simulink model "DTU_Topology_Medium_Line"  (R2023b)
settings: Solver=ode4  StartTime=0.0  StopTime=stoptime  FixedStep=Ts  RelTol=1e-3
PreLoadFcn:
  | Ts=1e-4;run('Grid_Parameters_3ph.m');load('Data_3ph_Pars.mat');load('First_Busbar_Pars.mat');load('PV_Busbar_Pars.mat');load('V2G_Busbar_Pars.mat');run('line_parameters.m')
PostLoadFcn:
  | Ts=1e-4;run('Grid_Parameters_3ph.m');load('Data_3ph_Pars.mat');load('First_Busbar_Pars.mat');load('PV_Busbar_Pars.mat');load('V2G_Busbar_Pars.mat');run('line_parameters.m')
InitFcn:
  | Ts=1e-4;run('Grid_Parameters_3ph.m');load('Data_3ph_Pars.mat');load('First_Busbar_Pars.mat');load('PV_Busbar_Pars.mat');load('V2G_Busbar_Pars.mat');run('line_parameters.m')
StartFcn:
  | Ts=1e-4;run('Grid_Parameters_3ph.m');load('Data_3ph_Pars.mat');load('First_Busbar_Pars.mat');load('PV_Busbar_Pars.mat');load('V2G_Busbar_Pars.mat');run('line_parameters.m')
values from neighbouring files (symbols this model uses):
  datastart = 6100    [Grid_Parameters_3ph.m]
  datastop = 6300    [Grid_Parameters_3ph.m]
  fnom = 50    [Grid_Parameters_3ph.m]    (also in line_parameters.m)
  line_param = struct()    [line_parameters.m]
  t_factor = 1/acceleration    (= 1)    [Grid_Parameters_3ph.m]
  timestep_meas_data = 1    [Grid_Parameters_3ph.m]
  Vnom = 400    [Grid_Parameters_3ph.m]
undefined symbols (not defined in the file or in its folder): another_event_name, Data_3ph_Pars, j, my_event_name, Newton, PV_Busbar_Pars, Raphson, V2G_Busbar_Pars
libraries: spsSeriesRLCBranchLib x57, spsGroundLib x30, spsThreePhaseVIMeasurementLib x17, spsControlledCurrentSourceLib x9, spsThreePhaseSineGeneratorLib x9, spsMeanLib x7, spsMutualInductanceLib x4, rtlab x2, spsThreePhaseSourceLib x1, sps_lib x1
(part 2 of 2)

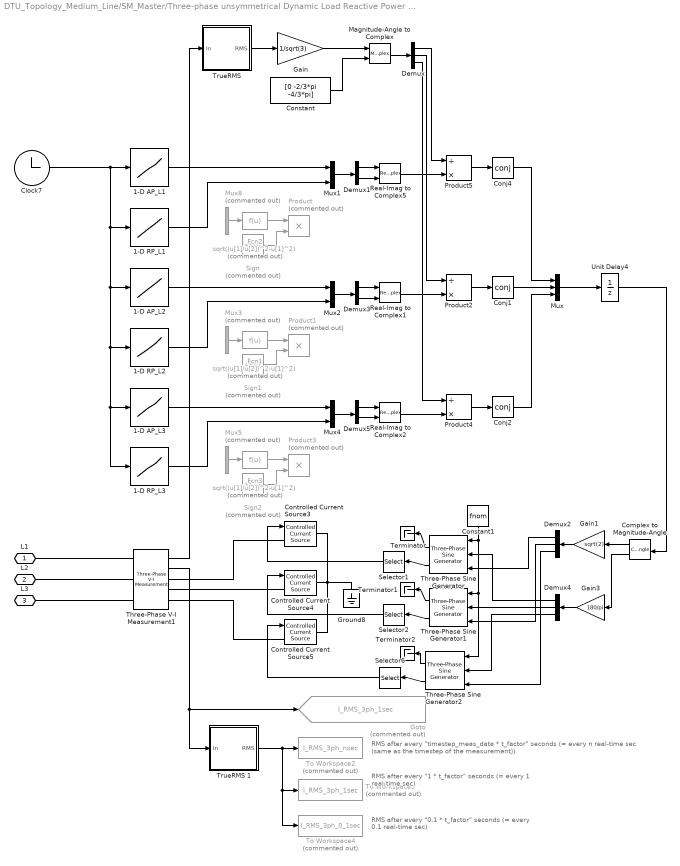
== system DTU_Topology_Medium_Line/SM_Master/Three-phase unsymmetrical Dynamic Load Reactive Power input PV ==
  note: RMS after every "1 * t_factor" seconds
      | (= every 1 real-time sec)
  note: RMS after every "0.1 * t_factor" seconds
      | (= every 0.1 real-time sec)
  note: RMS after every "timestep_meas_data * t_factor" seconds
      | (= every n real-time sec (same as the timestep of the measurement))
  1-D AP_L1 : Lookup_n-D  NumberOfTableDimensions=1  BreakpointsForDimension1=t_factor * [0:timestep_meas_data:(PV_Busbar_Pars.Time(datastop)-PV_Busbar_Pars.Time(datastart))]'  Table=PV_Busbar_Pars.ActivePowerL1(datastart:datastop)  InterpMethod=Flat  InternalRulePriority=Speed  RndMeth=Simplest
  1-D AP_L2 : Lookup_n-D  NumberOfTableDimensions=1  BreakpointsForDimension1=t_factor * [0:timestep_meas_data:(PV_Busbar_Pars.Time(datastop)-PV_Busbar_Pars.Time(datastart))]'  Table=PV_Busbar_Pars.ActivePowerL2(datastart:datastop)  InterpMethod=Flat  InternalRulePriority=Speed  RndMeth=Simplest
  1-D AP_L3 : Lookup_n-D  NumberOfTableDimensions=1  BreakpointsForDimension1=t_factor * [0:timestep_meas_data:(PV_Busbar_Pars.Time(datastop)-PV_Busbar_Pars.Time(datastart))]'  Table=PV_Busbar_Pars.ActivePowerL3(datastart:datastop)  InterpMethod=Flat  InternalRulePriority=Speed  RndMeth=Simplest
  1-D RP_L1 : Lookup_n-D  NumberOfTableDimensions=1  BreakpointsForDimension1=t_factor * [0:timestep_meas_data:(PV_Busbar_Pars.Time(datastop)-PV_Busbar_Pars.Time(datastart))]'  Table=PV_Busbar_Pars.ReactivePowerL1(datastart:datastop)  InterpMethod=Flat  InternalRulePriority=Speed  RndMeth=Simplest
  1-D RP_L2 : Lookup_n-D  NumberOfTableDimensions=1  BreakpointsForDimension1=t_factor * [0:timestep_meas_data:(PV_Busbar_Pars.Time(datastop)-PV_Busbar_Pars.Time(datastart))]'  Table=PV_Busbar_Pars.ReactivePowerL2(datastart:datastop)  InterpMethod=Flat  InternalRulePriority=Speed  RndMeth=Simplest
  1-D RP_L3 : Lookup_n-D  NumberOfTableDimensions=1  BreakpointsForDimension1=t_factor * [0:timestep_meas_data:(PV_Busbar_Pars.Time(datastop)-PV_Busbar_Pars.Time(datastart))]'  Table=PV_Busbar_Pars.ReactivePowerL3(datastart:datastop)  InterpMethod=Flat  InternalRulePriority=Speed  RndMeth=Simplest
  Clock7 : Clock
  Complex to Magnitude-Angle : ComplexToMagnitudeAngle
  Conj1 : Math  Operator=conj  SignedPower=on
  Conj2 : Math  Operator=conj  SignedPower=on
  Conj4 : Math  Operator=conj  SignedPower=on
  Constant : Constant  Value=[0 -2/3*pi -4/3*pi]
  Constant1 : Constant  Value=fnom
  Controlled Current Source3 : spsControlledCurrentSourceLib/Controlled Current Source  Initialize=on  Source_Type=AC  Amplitude=0  Phase=0  Frequency=50  Measurements=Current
  Controlled Current Source4 : spsControlledCurrentSourceLib/Controlled Current Source  Initialize=on  Source_Type=AC  Amplitude=0  Phase=0  Frequency=50  Measurements=Current
  Controlled Current Source5 : spsControlledCurrentSourceLib/Controlled Current Source  Initialize=on  Source_Type=AC  Amplitude=0  Phase=0  Frequency=50  Measurements=Current
  Demux : Demux  Outputs=3
  Demux1 : Demux  Outputs=2
      settings: DisplayOption=none
  Demux2 : Demux  Outputs=3
  Demux3 : Demux  Outputs=2
      settings: DisplayOption=none
  Demux4 : Demux  Outputs=3
  Demux5 : Demux  Outputs=2
      settings: DisplayOption=none
  Fcn1 : Fcn  Commented=on  Expr=sqrt((u[1]/u[2])^2-u[1]^2)
  Fcn2 : Fcn  Commented=on  Expr=sqrt((u[1]/u[2])^2-u[1]^2)
  Fcn3 : Fcn  Commented=on  Expr=sqrt((u[1]/u[2])^2-u[1]^2)
  Gain : Gain  Gain=1/sqrt(3)
  Gain1 : Gain  Gain=sqrt(2)
  Gain3 : Gain  Gain=180/pi
  Goto : Goto  Commented=on  GotoTag=I_RMS_3ph_1sec  TagVisibility=global
  Ground8 : spsGroundLib/Ground  LConnTagsString=a
  Magnitude-Angle to Complex : MagnitudeAngleToComplex
  Mux : Mux  Inputs=3
  Mux1 : Mux  Inputs=2
  Mux2 : Mux  Inputs=2
  Mux3 : Mux  Commented=on  Inputs=2
  Mux4 : Mux  Inputs=2
  Mux5 : Mux  Commented=on  Inputs=2
  Mux8 : Mux  Commented=on  Inputs=2
  Product : Product  Commented=on
  Product1 : Product  Commented=on
  Product2 : Product  Inputs=/*  InputSameDT=on  SaturateOnIntegerOverflow=on  OutDataTypeStr=Inherit: Same as first input
  Product3 : Product  Commented=on
  Product4 : Product  Inputs=/*  InputSameDT=on  SaturateOnIntegerOverflow=on  OutDataTypeStr=Inherit: Same as first input
  Product5 : Product  Inputs=/*  InputSameDT=on  SaturateOnIntegerOverflow=on  OutDataTypeStr=Inherit: Same as first input
  Real-Imag to Complex1 : RealImagToComplex
  Real-Imag to Complex2 : RealImagToComplex
  Real-Imag to Complex5 : RealImagToComplex
  Selector1 : Selector  InputPortWidth=3  IndexOptions=Index vector (dialog)  Indices=1  OutputSizes=1
  Selector2 : Selector  InputPortWidth=3  IndexOptions=Index vector (dialog)  Indices=1  OutputSizes=1
  Selector6 : Selector  InputPortWidth=3  IndexOptions=Index vector (dialog)  Indices=1  OutputSizes=1
  Sign : Signum  Commented=on
  Sign1 : Signum  Commented=on
  Sign2 : Signum  Commented=on
  Terminator : Terminator
  Terminator1 : Terminator
  Terminator2 : Terminator
  Three-Phase Sine Generator : spsThreePhaseSineGeneratorLib/Three-Phase Sine Generator  Ts=0
      settings: LibrarySourceBlock=|
      | sps_lib/Sources/Signal Generator Sources/Three-Phase
      | Sine Generator
  Three-Phase Sine Generator1 : spsThreePhaseSineGeneratorLib/Three-Phase Sine Generator  Ts=0
      settings: LibrarySourceBlock=|
      | sps_lib/Sources/Signal Generator Sources/Three-Phase
      | Sine Generator
  Three-Phase Sine Generator2 : spsThreePhaseSineGeneratorLib/Three-Phase Sine Generator  Ts=0
      settings: LibrarySourceBlock=|
      | sps_lib/Sources/Signal Generator Sources/Three-Phase
      | Sine Generator
  Three-Phase V-I Measurement1 : spsThreePhaseVIMeasurementLib/Three-Phase V-I Measurement  VoltageMeasurement=phase-to-phase  SetLabelV=off  LabelV=Vabc  Vpu=off  VpuLL=off  CurrentMeasurement=yes  SetLabelI=off  LabelI=Iabc  Ipu=off  Pbase=100e6  Vbase=Vnom*sqrt(3)  OutputType=Complex  PhasorSimulation=off  PSBequivalent=0
  To Workspace2 : ToWorkspace  Commented=on  VariableName=I_RMS_3ph_nsec  SampleTime=timestep_meas_data * t_factor
  To Workspace4 : ToWorkspace  Commented=on  VariableName=I_RMS_3ph_0_1sec  SampleTime=0.1 * t_factor
  To Workspace5 : ToWorkspace  Commented=on  VariableName=I_RMS_3ph_1sec  SampleTime=1 * t_factor
  "TrueRMS " : Subsystem  AncestorBlock=powerlib_meascontrol/Measurements/RMS/TrueRMS
  TrueRMS 1 : Subsystem  AncestorBlock=powerlib_meascontrol/Measurements/RMS/TrueRMS
  Unit Delay4 : UnitDelay  InitialCondition=0*exp(-j*0*pi/180)  SampleTime=Ts  HasFrameUpgradeWarning=on
  L1 : PMIOPort  Side=Right
  L2 : PMIOPort  Port=2  Side=Right
  L3 : PMIOPort  Port=3  Side=Right
  wires:
  1-D AP_L1/1 -> Mux1/1
  Product5/1 -> Conj4/1
  Fcn2/1 -> Product/1
  Three-Phase V-I Measurement1/2 -> Goto/1, TrueRMS 1/1(In)
  Mux1/1 -> Demux1/1
  Real-Imag to Complex5/1 -> Product5/2
  Clock7/1 -> 1-D RP_L1/1, 1-D RP_L2/1, 1-D AP_L3/1, 1-D RP_L3/1, 1-D AP_L2/1, 1-D AP_L1/1
  Sign/1 -> Product/2
  Mux8/1 -> Fcn2/1
  TrueRMS 1/1(RMS) -> To Workspace2/1, To Workspace5/1, To Workspace4/1
  Constant/1 -> Magnitude-Angle to Complex/2
  Demux/1 -> Product5/1
  Demux/2 -> Product2/1
  Demux/3 -> Product4/1
  Magnitude-Angle to Complex/1 -> Demux/1
  Gain/1 -> Magnitude-Angle to Complex/1
  Mux/1 -> Unit Delay4/1
  Complex to Magnitude-Angle/1 -> Gain1/1
  Three-Phase Sine Generator/1 -> Selector1/1
  Three-Phase Sine Generator1/1 -> Selector2/1
  Three-Phase Sine Generator2/1 -> Selector6/1
  Selector2/1 -> Controlled Current Source4/1
  Selector6/1 -> Controlled Current Source5/1
  Demux2/1 -> Three-Phase Sine Generator/1
  Demux2/2 -> Three-Phase Sine Generator1/1
  Demux2/3 -> Three-Phase Sine Generator2/1
  Conj4/1 -> Mux/1
  Conj1/1 -> Mux/2
  Conj2/1 -> Mux/3
  Constant1/1 -> Three-Phase Sine Generator/3, Three-Phase Sine Generator2/3, Three-Phase Sine Generator1/3
  Complex to Magnitude-Angle/2 -> Gain3/1
  Gain3/1 -> Demux4/1
  Selector1/1 -> Controlled Current Source3/1
  Demux4/1 -> Three-Phase Sine Generator/2
  Demux4/2 -> Three-Phase Sine Generator1/2
  Demux4/3 -> Three-Phase Sine Generator2/2
  Gain1/1 -> Demux2/1
  Demux1/1 -> Real-Imag to Complex5/1
  Demux1/2 -> Real-Imag to Complex5/2
  "TrueRMS "/1(RMS) -> Gain/1
  Three-Phase V-I Measurement1/1 -> "TrueRMS "/1(In)
  Unit Delay4/1 -> Complex to Magnitude-Angle/1
  Mux2/1 -> Demux3/1
  Demux3/2 -> Real-Imag to Complex1/2
  Real-Imag to Complex1/1 -> Product2/2
  Sign1/1 -> Product1/2
  Demux3/1 -> Real-Imag to Complex1/1
  Mux3/1 -> Fcn1/1
  1-D AP_L2/1 -> Mux2/1
  Product2/1 -> Conj1/1
  Fcn1/1 -> Product1/1
  Mux4/1 -> Demux5/1
  Demux5/2 -> Real-Imag to Complex2/2
  Real-Imag to Complex2/1 -> Product4/2
  Sign2/1 -> Product3/2
  Demux5/1 -> Real-Imag to Complex2/1
  Mux5/1 -> Fcn3/1
  1-D AP_L3/1 -> Mux4/1
  Product4/1 -> Conj2/1
  Fcn3/1 -> Product3/1
  1-D RP_L1/1 -> Mux1/2
  1-D RP_L2/1 -> Mux2/2
  1-D RP_L3/1 -> Mux4/2
  Three-Phase Sine Generator/2 -> Terminator/1
  Three-Phase Sine Generator1/2 -> Terminator1/1
  Three-Phase Sine Generator2/2 -> Terminator2/1
  connections:
  Three-Phase V-I Measurement1/RConn2 -- Controlled Current Source4/LConn1
  Three-Phase V-I Measurement1/RConn1 -- Controlled Current Source3/LConn1
  Three-Phase V-I Measurement1/RConn3 -- Controlled Current Source5/LConn1
  Controlled Current Source3/RConn1 -- Controlled Current Source4/RConn1 -- Ground8/LConn1 -- Controlled Current Source5/RConn1
  L1/RConn1 -- Three-Phase V-I Measurement1/LConn1
  Three-Phase V-I Measurement1/LConn2 -- L2/RConn1
  Three-Phase V-I Measurement1/LConn3 -- L3/RConn1

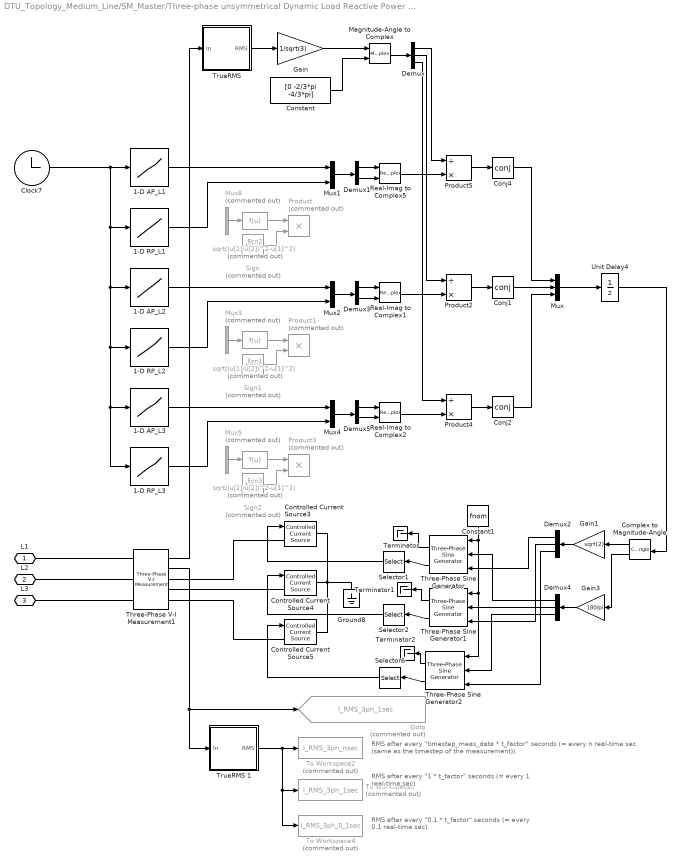
== system DTU_Topology_Medium_Line/SM_Master/Three-phase unsymmetrical Dynamic Load Reactive Power input V2G ==
  note: RMS after every "1 * t_factor" seconds
      | (= every 1 real-time sec)
  note: RMS after every "0.1 * t_factor" seconds
      | (= every 0.1 real-time sec)
  note: RMS after every "timestep_meas_data * t_factor" seconds
      | (= every n real-time sec (same as the timestep of the measurement))
  1-D AP_L1 : Lookup_n-D  NumberOfTableDimensions=1  BreakpointsForDimension1=t_factor * [0:timestep_meas_data:(V2G_Busbar_Pars.Time(datastop)-V2G_Busbar_Pars.Time(datastart))]'  Table=V2G_Busbar_Pars.ActivePowerL1(datastart:datastop)  InterpMethod=Flat  InternalRulePriority=Speed  RndMeth=Simplest
  1-D AP_L2 : Lookup_n-D  NumberOfTableDimensions=1  BreakpointsForDimension1=t_factor * [0:timestep_meas_data:(V2G_Busbar_Pars.Time(datastop)-V2G_Busbar_Pars.Time(datastart))]'  Table=V2G_Busbar_Pars.ActivePowerL2(datastart:datastop)  InterpMethod=Flat  InternalRulePriority=Speed  RndMeth=Simplest
  1-D AP_L3 : Lookup_n-D  NumberOfTableDimensions=1  BreakpointsForDimension1=t_factor * [0:timestep_meas_data:(V2G_Busbar_Pars.Time(datastop)-V2G_Busbar_Pars.Time(datastart))]'  Table=V2G_Busbar_Pars.ActivePowerL3(datastart:datastop)  InterpMethod=Flat  InternalRulePriority=Speed  RndMeth=Simplest
  1-D RP_L1 : Lookup_n-D  NumberOfTableDimensions=1  BreakpointsForDimension1=t_factor * [0:timestep_meas_data:(V2G_Busbar_Pars.Time(datastop)-V2G_Busbar_Pars.Time(datastart))]'  Table=V2G_Busbar_Pars.ReactivePowerL1(datastart:datastop)  InterpMethod=Flat  InternalRulePriority=Speed  RndMeth=Simplest
  1-D RP_L2 : Lookup_n-D  NumberOfTableDimensions=1  BreakpointsForDimension1=t_factor * [0:timestep_meas_data:(V2G_Busbar_Pars.Time(datastop)-V2G_Busbar_Pars.Time(datastart))]'  Table=V2G_Busbar_Pars.ReactivePowerL2(datastart:datastop)  InterpMethod=Flat  InternalRulePriority=Speed  RndMeth=Simplest
  1-D RP_L3 : Lookup_n-D  NumberOfTableDimensions=1  BreakpointsForDimension1=t_factor * [0:timestep_meas_data:(V2G_Busbar_Pars.Time(datastop)-V2G_Busbar_Pars.Time(datastart))]'  Table=V2G_Busbar_Pars.ReactivePowerL3(datastart:datastop)  InterpMethod=Flat  InternalRulePriority=Speed  RndMeth=Simplest
  Clock7 : Clock
  Complex to Magnitude-Angle : ComplexToMagnitudeAngle
  Conj1 : Math  Operator=conj  SignedPower=on
  Conj2 : Math  Operator=conj  SignedPower=on
  Conj4 : Math  Operator=conj  SignedPower=on
  Constant : Constant  Value=[0 -2/3*pi -4/3*pi]
  Constant1 : Constant  Value=fnom
  Controlled Current Source3 : spsControlledCurrentSourceLib/Controlled Current Source  Initialize=on  Source_Type=AC  Amplitude=0  Phase=0  Frequency=50  Measurements=Current
  Controlled Current Source4 : spsControlledCurrentSourceLib/Controlled Current Source  Initialize=on  Source_Type=AC  Amplitude=0  Phase=0  Frequency=50  Measurements=Current
  Controlled Current Source5 : spsControlledCurrentSourceLib/Controlled Current Source  Initialize=on  Source_Type=AC  Amplitude=0  Phase=0  Frequency=50  Measurements=Current
  Demux : Demux  Outputs=3
  Demux1 : Demux  Outputs=2
      settings: DisplayOption=none
  Demux2 : Demux  Outputs=3
  Demux3 : Demux  Outputs=2
      settings: DisplayOption=none
  Demux4 : Demux  Outputs=3
  Demux5 : Demux  Outputs=2
      settings: DisplayOption=none
  Fcn1 : Fcn  Commented=on  Expr=sqrt((u[1]/u[2])^2-u[1]^2)
  Fcn2 : Fcn  Commented=on  Expr=sqrt((u[1]/u[2])^2-u[1]^2)
  Fcn3 : Fcn  Commented=on  Expr=sqrt((u[1]/u[2])^2-u[1]^2)
  Gain : Gain  Gain=1/sqrt(3)
  Gain1 : Gain  Gain=sqrt(2)
  Gain3 : Gain  Gain=180/pi
  Goto : Goto  Commented=on  GotoTag=I_RMS_3ph_1sec  TagVisibility=global
  Ground8 : spsGroundLib/Ground  LConnTagsString=a
  Magnitude-Angle to Complex : MagnitudeAngleToComplex
  Mux : Mux  Inputs=3
  Mux1 : Mux  Inputs=2
  Mux2 : Mux  Inputs=2
  Mux3 : Mux  Commented=on  Inputs=2
  Mux4 : Mux  Inputs=2
  Mux5 : Mux  Commented=on  Inputs=2
  Mux8 : Mux  Commented=on  Inputs=2
  Product : Product  Commented=on
  Product1 : Product  Commented=on
  Product2 : Product  Inputs=/*  InputSameDT=on  SaturateOnIntegerOverflow=on  OutDataTypeStr=Inherit: Same as first input
  Product3 : Product  Commented=on
  Product4 : Product  Inputs=/*  InputSameDT=on  SaturateOnIntegerOverflow=on  OutDataTypeStr=Inherit: Same as first input
  Product5 : Product  Inputs=/*  InputSameDT=on  SaturateOnIntegerOverflow=on  OutDataTypeStr=Inherit: Same as first input
  Real-Imag to Complex1 : RealImagToComplex
  Real-Imag to Complex2 : RealImagToComplex
  Real-Imag to Complex5 : RealImagToComplex
  Selector1 : Selector  InputPortWidth=3  IndexOptions=Index vector (dialog)  Indices=1  OutputSizes=1
  Selector2 : Selector  InputPortWidth=3  IndexOptions=Index vector (dialog)  Indices=1  OutputSizes=1
  Selector6 : Selector  InputPortWidth=3  IndexOptions=Index vector (dialog)  Indices=1  OutputSizes=1
  Sign : Signum  Commented=on
  Sign1 : Signum  Commented=on
  Sign2 : Signum  Commented=on
  Terminator : Terminator
  Terminator1 : Terminator
  Terminator2 : Terminator
  Three-Phase Sine Generator : spsThreePhaseSineGeneratorLib/Three-Phase Sine Generator  Ts=0
      settings: LibrarySourceBlock=|
      | sps_lib/Sources/Signal Generator Sources/Three-Phase
      | Sine Generator
  Three-Phase Sine Generator1 : spsThreePhaseSineGeneratorLib/Three-Phase Sine Generator  Ts=0
      settings: LibrarySourceBlock=|
      | sps_lib/Sources/Signal Generator Sources/Three-Phase
      | Sine Generator
  Three-Phase Sine Generator2 : spsThreePhaseSineGeneratorLib/Three-Phase Sine Generator  Ts=0
      settings: LibrarySourceBlock=|
      | sps_lib/Sources/Signal Generator Sources/Three-Phase
      | Sine Generator
  Three-Phase V-I Measurement1 : spsThreePhaseVIMeasurementLib/Three-Phase V-I Measurement  VoltageMeasurement=phase-to-phase  SetLabelV=off  LabelV=Vabc  Vpu=off  VpuLL=off  CurrentMeasurement=yes  SetLabelI=off  LabelI=Iabc  Ipu=off  Pbase=100e6  Vbase=Vnom*sqrt(3)  OutputType=Complex  PhasorSimulation=off  PSBequivalent=0
  To Workspace2 : ToWorkspace  Commented=on  VariableName=I_RMS_3ph_nsec  SampleTime=timestep_meas_data * t_factor
  To Workspace4 : ToWorkspace  Commented=on  VariableName=I_RMS_3ph_0_1sec  SampleTime=0.1 * t_factor
  To Workspace5 : ToWorkspace  Commented=on  VariableName=I_RMS_3ph_1sec  SampleTime=1 * t_factor
  "TrueRMS " : Subsystem  AncestorBlock=powerlib_meascontrol/Measurements/RMS/TrueRMS
  TrueRMS 1 : Subsystem  AncestorBlock=powerlib_meascontrol/Measurements/RMS/TrueRMS
  Unit Delay4 : UnitDelay  InitialCondition=0*exp(-j*0*pi/180)  SampleTime=Ts  HasFrameUpgradeWarning=on
  L1 : PMIOPort  Side=Right
  L2 : PMIOPort  Port=2  Side=Right
  L3 : PMIOPort  Port=3  Side=Right
  wires:
  1-D AP_L1/1 -> Mux1/1
  Product5/1 -> Conj4/1
  Fcn2/1 -> Product/1
  Three-Phase V-I Measurement1/2 -> Goto/1, TrueRMS 1/1(In)
  Mux1/1 -> Demux1/1
  Real-Imag to Complex5/1 -> Product5/2
  Clock7/1 -> 1-D RP_L1/1, 1-D RP_L2/1, 1-D AP_L3/1, 1-D RP_L3/1, 1-D AP_L2/1, 1-D AP_L1/1
  Sign/1 -> Product/2
  Mux8/1 -> Fcn2/1
  TrueRMS 1/1(RMS) -> To Workspace2/1, To Workspace5/1, To Workspace4/1
  Constant/1 -> Magnitude-Angle to Complex/2
  Demux/1 -> Product5/1
  Demux/2 -> Product2/1
  Demux/3 -> Product4/1
  Magnitude-Angle to Complex/1 -> Demux/1
  Gain/1 -> Magnitude-Angle to Complex/1
  Mux/1 -> Unit Delay4/1
  Complex to Magnitude-Angle/1 -> Gain1/1
  Three-Phase Sine Generator/1 -> Selector1/1
  Three-Phase Sine Generator1/1 -> Selector2/1
  Three-Phase Sine Generator2/1 -> Selector6/1
  Selector2/1 -> Controlled Current Source4/1
  Selector6/1 -> Controlled Current Source5/1
  Demux2/1 -> Three-Phase Sine Generator/1
  Demux2/2 -> Three-Phase Sine Generator1/1
  Demux2/3 -> Three-Phase Sine Generator2/1
  Conj4/1 -> Mux/1
  Conj1/1 -> Mux/2
  Conj2/1 -> Mux/3
  Constant1/1 -> Three-Phase Sine Generator/3, Three-Phase Sine Generator2/3, Three-Phase Sine Generator1/3
  Complex to Magnitude-Angle/2 -> Gain3/1
  Gain3/1 -> Demux4/1
  Selector1/1 -> Controlled Current Source3/1
  Demux4/1 -> Three-Phase Sine Generator/2
  Demux4/2 -> Three-Phase Sine Generator1/2
  Demux4/3 -> Three-Phase Sine Generator2/2
  Gain1/1 -> Demux2/1
  Demux1/1 -> Real-Imag to Complex5/1
  Demux1/2 -> Real-Imag to Complex5/2
  "TrueRMS "/1(RMS) -> Gain/1
  Three-Phase V-I Measurement1/1 -> "TrueRMS "/1(In)
  Unit Delay4/1 -> Complex to Magnitude-Angle/1
  Mux2/1 -> Demux3/1
  Demux3/2 -> Real-Imag to Complex1/2
  Real-Imag to Complex1/1 -> Product2/2
  Sign1/1 -> Product1/2
  Demux3/1 -> Real-Imag to Complex1/1
  Mux3/1 -> Fcn1/1
  1-D AP_L2/1 -> Mux2/1
  Product2/1 -> Conj1/1
  Fcn1/1 -> Product1/1
  Mux4/1 -> Demux5/1
  Demux5/2 -> Real-Imag to Complex2/2
  Real-Imag to Complex2/1 -> Product4/2
  Sign2/1 -> Product3/2
  Demux5/1 -> Real-Imag to Complex2/1
  Mux5/1 -> Fcn3/1
  1-D AP_L3/1 -> Mux4/1
  Product4/1 -> Conj2/1
  Fcn3/1 -> Product3/1
  1-D RP_L1/1 -> Mux1/2
  1-D RP_L2/1 -> Mux2/2
  1-D RP_L3/1 -> Mux4/2
  Three-Phase Sine Generator/2 -> Terminator/1
  Three-Phase Sine Generator1/2 -> Terminator1/1
  Three-Phase Sine Generator2/2 -> Terminator2/1
  connections:
  Three-Phase V-I Measurement1/RConn2 -- Controlled Current Source4/LConn1
  Three-Phase V-I Measurement1/RConn1 -- Controlled Current Source3/LConn1
  Three-Phase V-I Measurement1/RConn3 -- Controlled Current Source5/LConn1
  Controlled Current Source3/RConn1 -- Controlled Current Source4/RConn1 -- Ground8/LConn1 -- Controlled Current Source5/RConn1
  L1/RConn1 -- Three-Phase V-I Measurement1/LConn1
  Three-Phase V-I Measurement1/LConn2 -- L2/RConn1
  Three-Phase V-I Measurement1/LConn3 -- L3/RConn1

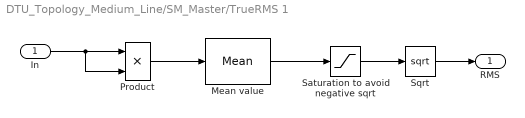
== system DTU_Topology_Medium_Line/SM_Master/TrueRMS 1 ==
  In : Inport
  Mean value : spsMeanLib/Mean  Freq=fnom  Vinit=0  Ts=Ts
  Product : Product  InputSameDT=on  SaturateOnIntegerOverflow=on  OutDataTypeStr=Inherit: Same as first input
  Saturation to avoid negative sqrt : Saturate  UpperLimit=Inf  LowerLimit=0
  Sqrt : Sqrt  AlgorithmType=Newton-Raphson
  RMS : Outport  VectorParamsAs1DForOutWhenUnconnected=off
  wires:
  Saturation to avoid negative sqrt/1 -> Sqrt/1
  Mean value/1 -> Saturation to avoid negative sqrt/1
  Product/1 -> Mean value/1
  In/1 -> Product/2, Product/1
  Sqrt/1 -> RMS/1

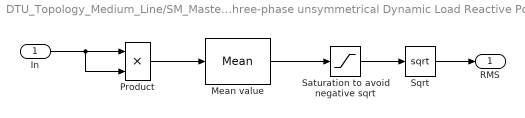
== system DTU_Topology_Medium_Line/SM_Master/Three-phase unsymmetrical Dynamic Load Reactive Power input Dump load/TrueRMS  ==
  In : Inport
  Mean value : spsMeanLib/Mean  Freq=fnom  Vinit=400^2  Ts=Ts
  Product : Product  InputSameDT=on  SaturateOnIntegerOverflow=on  OutDataTypeStr=Inherit: Same as first input
  Saturation to avoid negative sqrt : Saturate  UpperLimit=Inf  LowerLimit=0
  Sqrt : Sqrt  AlgorithmType=Newton-Raphson
  RMS : Outport  VectorParamsAs1DForOutWhenUnconnected=off
  wires:
  Saturation to avoid negative sqrt/1 -> Sqrt/1
  Mean value/1 -> Saturation to avoid negative sqrt/1
  Product/1 -> Mean value/1
  In/1 -> Product/2, Product/1
  Sqrt/1 -> RMS/1

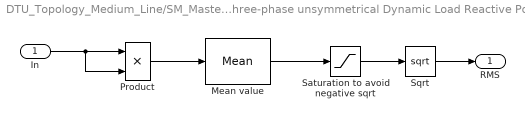
== system DTU_Topology_Medium_Line/SM_Master/Three-phase unsymmetrical Dynamic Load Reactive Power input Dump load/TrueRMS 1 ==
  In : Inport
  Mean value : spsMeanLib/Mean  Freq=fnom  Vinit=0  Ts=Ts
  Product : Product  InputSameDT=on  SaturateOnIntegerOverflow=on  OutDataTypeStr=Inherit: Same as first input
  Saturation to avoid negative sqrt : Saturate  UpperLimit=Inf  LowerLimit=0
  Sqrt : Sqrt  AlgorithmType=Newton-Raphson
  RMS : Outport  VectorParamsAs1DForOutWhenUnconnected=off
  wires:
  Saturation to avoid negative sqrt/1 -> Sqrt/1
  Mean value/1 -> Saturation to avoid negative sqrt/1
  Product/1 -> Mean value/1
  In/1 -> Product/2, Product/1
  Sqrt/1 -> RMS/1

== system DTU_Topology_Medium_Line/SM_Master/Three-phase unsymmetrical Dynamic Load Reactive Power input PV/TrueRMS  ==
  In : Inport
  Mean value : spsMeanLib/Mean  Freq=fnom  Vinit=400^2  Ts=Ts
  Product : Product  InputSameDT=on  SaturateOnIntegerOverflow=on  OutDataTypeStr=Inherit: Same as first input
  Saturation to avoid negative sqrt : Saturate  UpperLimit=Inf  LowerLimit=0
  Sqrt : Sqrt  AlgorithmType=Newton-Raphson
  RMS : Outport  VectorParamsAs1DForOutWhenUnconnected=off
  wires:
  Saturation to avoid negative sqrt/1 -> Sqrt/1
  Mean value/1 -> Saturation to avoid negative sqrt/1
  Product/1 -> Mean value/1
  In/1 -> Product/2, Product/1
  Sqrt/1 -> RMS/1

== system DTU_Topology_Medium_Line/SM_Master/Three-phase unsymmetrical Dynamic Load Reactive Power input PV/TrueRMS 1 ==
  In : Inport
  Mean value : spsMeanLib/Mean  Freq=fnom  Vinit=0  Ts=Ts
  Product : Product  InputSameDT=on  SaturateOnIntegerOverflow=on  OutDataTypeStr=Inherit: Same as first input
  Saturation to avoid negative sqrt : Saturate  UpperLimit=Inf  LowerLimit=0
  Sqrt : Sqrt  AlgorithmType=Newton-Raphson
  RMS : Outport  VectorParamsAs1DForOutWhenUnconnected=off
  wires:
  Saturation to avoid negative sqrt/1 -> Sqrt/1
  Mean value/1 -> Saturation to avoid negative sqrt/1
  Product/1 -> Mean value/1
  In/1 -> Product/2, Product/1
  Sqrt/1 -> RMS/1

== system DTU_Topology_Medium_Line/SM_Master/Three-phase unsymmetrical Dynamic Load Reactive Power input V2G/TrueRMS  ==
  In : Inport
  Mean value : spsMeanLib/Mean  Freq=fnom  Vinit=400^2  Ts=Ts
  Product : Product  InputSameDT=on  SaturateOnIntegerOverflow=on  OutDataTypeStr=Inherit: Same as first input
  Saturation to avoid negative sqrt : Saturate  UpperLimit=Inf  LowerLimit=0
  Sqrt : Sqrt  AlgorithmType=Newton-Raphson
  RMS : Outport  VectorParamsAs1DForOutWhenUnconnected=off
  wires:
  Saturation to avoid negative sqrt/1 -> Sqrt/1
  Mean value/1 -> Saturation to avoid negative sqrt/1
  Product/1 -> Mean value/1
  In/1 -> Product/2, Product/1
  Sqrt/1 -> RMS/1

== system DTU_Topology_Medium_Line/SM_Master/Three-phase unsymmetrical Dynamic Load Reactive Power input V2G/TrueRMS 1 ==
  In : Inport
  Mean value : spsMeanLib/Mean  Freq=fnom  Vinit=0  Ts=Ts
  Product : Product  InputSameDT=on  SaturateOnIntegerOverflow=on  OutDataTypeStr=Inherit: Same as first input
  Saturation to avoid negative sqrt : Saturate  UpperLimit=Inf  LowerLimit=0
  Sqrt : Sqrt  AlgorithmType=Newton-Raphson
  RMS : Outport  VectorParamsAs1DForOutWhenUnconnected=off
  wires:
  Saturation to avoid negative sqrt/1 -> Sqrt/1
  Mean value/1 -> Saturation to avoid negative sqrt/1
  Product/1 -> Mean value/1
  In/1 -> Product/2, Product/1
  Sqrt/1 -> RMS/1
